simulink model "string2"  (R2018b)
settings: Solver=VariableStepAuto  StartTime=0.0  StopTime=10.0  RelTol=1e-3
libraries: powerlib x14, powerlib_meascontrol x4
settings Model: Creator=HP  LastModifiedBy=HP

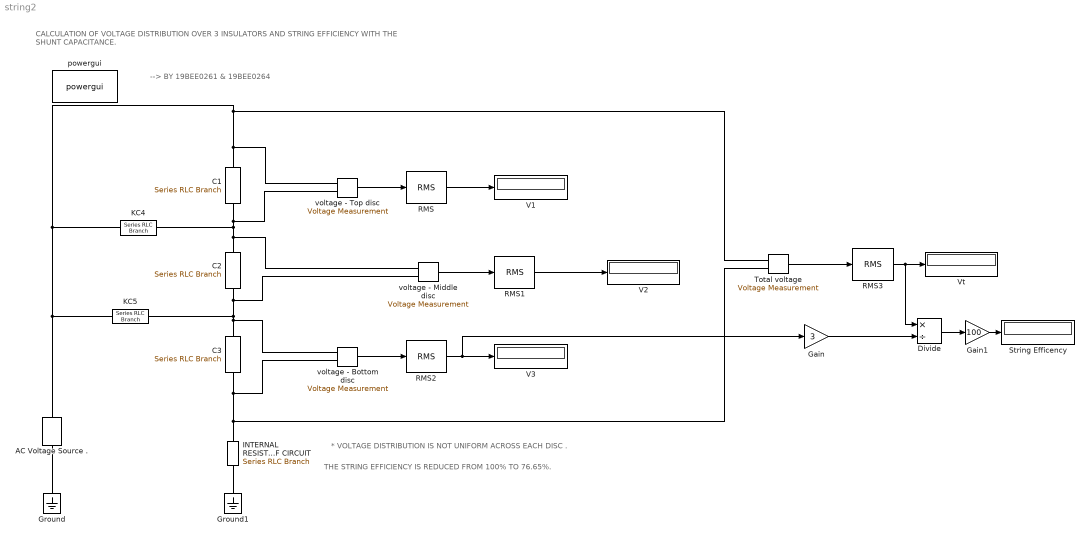
== system string2 ==
  note: THE STRING EFFICIENCY IS REDUCED FROM 100% TO 76.65%.
  note: * VOLTAGE DISTRIBUTION IS NOT UNIFORM ACROSS EACH DISC .
  note: --> BY 19BEE0261 & 19BEE0264
  note: CALCULATION OF VOLTAGE DISTRIBUTION OVER 3 INSULATORS AND STRING EFFICIENCY
      | WITH THE SHUNT CAPACITANCE.
  " Total voltage " : powerlib/Measurements/Voltage Measurement  PhasorSimulation=off  OutputType=Complex  PSBequivalent=0
  AC Voltage Source . : powerlib/Electrical Sources/AC Voltage Source  Amplitude=1.414*19.05*10^3  Phase=0  Frequency=60  SampleTime=0  Measurements=None  BusType=swing  Pref=10e3  Qref=0  Qmin=-inf  Qmax=+inf
  C1 : powerlib/Elements/Series RLC Branch  LConnTagsString=__new0  RConnTagsString=__new0  BranchType=C  Resistance=1  Inductance=1e-3  SetiL0=off  InitialCurrent=0  Capacitance=1e-6  Setx0=off  InitialVoltage=0  Measurements=None
  C2 : powerlib/Elements/Series RLC Branch  LConnTagsString=__new0  RConnTagsString=__new0  BranchType=C  Resistance=1  Inductance=1e-3  SetiL0=off  InitialCurrent=0  Capacitance=1e-6  Setx0=off  InitialVoltage=0  Measurements=None
  C3 : powerlib/Elements/Series RLC Branch  LConnTagsString=__new0  RConnTagsString=__new0  BranchType=C  Resistance=1  Inductance=1e-3  SetiL0=off  InitialCurrent=0  Capacitance=1e-6  Setx0=off  InitialVoltage=0  Measurements=None
  Divide : Product  Inputs=*/
  Gain : Gain  Gain=3
  Gain1 : Gain  Gain=100
  Ground : powerlib/Elements/Ground  LConnTagsString=a
  Ground1 : powerlib/Elements/Ground  LConnTagsString=a
  "INTERNAL RESISTANCE OF CIRCUIT " : powerlib/Elements/Series RLC Branch  LConnTagsString=__new0  RConnTagsString=__new0  BranchType=R  Resistance=1  Inductance=1e-3  SetiL0=off  InitialCurrent=0  Capacitance=1e-6  Setx0=off  InitialVoltage=0  Measurements=None
  KC4 : powerlib/Elements/Series RLC Branch  LConnTagsString=__new0  RConnTagsString=__new0  BranchType=C  Resistance=1  Inductance=1e-3  SetiL0=off  InitialCurrent=0  Capacitance=0.22e-6  Setx0=off  InitialVoltage=0  Measurements=None
  KC5 : powerlib/Elements/Series RLC Branch  LConnTagsString=__new0  RConnTagsString=__new0  BranchType=C  Resistance=1  Inductance=1e-3  SetiL0=off  InitialCurrent=0  Capacitance=0.22e-6  Setx0=off  InitialVoltage=0  Measurements=None
  RMS{,1..3} (4 alike) : powerlib_meascontrol/Measurements/RMS  TrueRMS=on  Freq=60  RMSInit=0  Ts=0
  String Efficency : Display
  V1 : Display
  V2 : Display
  V3 : Display
  Vt : Display
  powergui : powerlib/powergui  Priority=1  SimulationMode=Continuous  SampleTime=50e-6  frequency=60  Iterations=50  frequencyindice=60  Pbase=100e6  ErrMax=1e-4  UnitsV=kV  UnitsW=MW  buscounter=0  FunctionMessages=off  echomessages=off  EnableUseOfTLC=off  CurrentSourceSwitches=off  DisableSnubberDevices=off  DisableRonSwitches=off  DisableVfSwitches=off  DisplayEquations=off  SolverType=Tustin/Backward Euler (TBE)  Interpol=off  ExternalGateDelay=off  methode=off  Ts=100  x0status=blocks  SPID=on  SwTol=0  HookPort=off  RestoreLinks=warning  ResistiveCurrentMeasurement=off  Frange=[0:2:500]  Ylog=off  Xlog=on  ShowGrid=off  save=off  variable=ZData  structure=0  ZoomFFT=off  StartTime=0.0  cycles=1  DisplayStyle=1  fundamental=60  FreqAxis=off  MaxFrequency=1000  frequencyindicesteady=1  RmsSteady=1  display=off
  voltage - Bottom disc : powerlib/Measurements/Voltage Measurement  PhasorSimulation=off  OutputType=Complex  PSBequivalent=0
  voltage - Middle disc : powerlib/Measurements/Voltage Measurement  PhasorSimulation=off  OutputType=Complex  PSBequivalent=0
  voltage - Top disc : powerlib/Measurements/Voltage Measurement  PhasorSimulation=off  OutputType=Complex  PSBequivalent=0
  wires:
  Gain1/1 -> String Efficency/1
  " Total voltage "/1 -> RMS3/1
  voltage - Middle disc/1 -> RMS1/1
  Divide/1 -> Gain1/1
  RMS2/1 -> Gain/1, V3/1
  Gain/1 -> Divide/2
  RMS3/1 -> Divide/1, Vt/1
  RMS/1 -> V1/1
  RMS1/1 -> V2/1
  voltage - Top disc/1 -> RMS/1
  voltage - Bottom disc/1 -> RMS2/1
  connections:
  "INTERNAL RESISTANCE OF CIRCUIT "/LConn1 -- voltage - Bottom disc/LConn2 -- C3/RConn1 -- " Total voltage "/LConn2
  C2/RConn1 -- KC5/LConn1 -- C3/LConn1 -- voltage - Bottom disc/LConn1 -- voltage - Middle disc/LConn2
  C1/LConn1 -- KC5/RConn1 -- AC Voltage Source ./RConn1 -- KC4/RConn1 -- " Total voltage "/LConn1 -- voltage - Top disc/LConn1
  C1/RConn1 -- KC4/LConn1 -- C2/LConn1 -- voltage - Middle disc/LConn1 -- voltage - Top disc/LConn2
  "INTERNAL RESISTANCE OF CIRCUIT "/RConn1 -- Ground1/LConn1
  Ground/LConn1 -- AC Voltage Source ./LConn1
